simulink model "shit"  (R2019b)
settings: Solver=VariableStepAuto  StartTime=0.0  StopTime=10.0  RelTol=1e-3
libraries: simulink x2
settings Model: Creator=kWX1197707  LastModifiedBy=kWX1197707

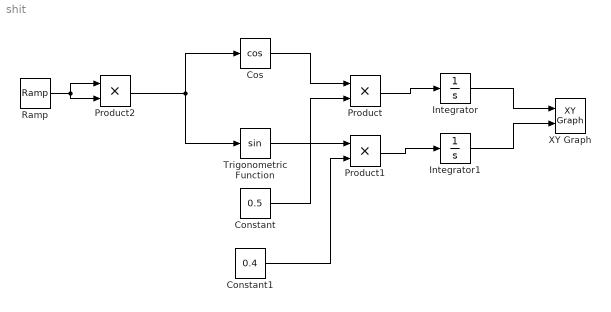
== system shit ==
  Constant : Constant  Value=0.5
  Constant1 : Constant  Value=0.4
  Cos : Trigonometry  Operator=cos
  Integrator : Integrator
  Integrator1 : Integrator
  Product : Product
  Product1 : Product
  Product2 : Product
  Ramp : simulink/Sources/Ramp  slope=1  start=0  InitialOutput=0
  Trigonometric Function : Trigonometry
  XY Graph : simulink/Sinks/XY Graph  xmin=-1  xmax=1  ymin=-1  ymax=1  st=-1
  wires:
  Trigonometric Function/1 -> Product1/1
  Cos/1 -> Product/1
  Ramp/1 -> Product2/2, Product2/1
  Product/1 -> Integrator/1
  Product1/1 -> Integrator1/1
  Integrator1/1 -> XY Graph/2
  Integrator/1 -> XY Graph/1
  Product2/1 -> Cos/1, Trigonometric Function/1
  Constant/1 -> Product/2
  Constant1/1 -> Product1/2
